simulink model "controller"  (Simulink 8.7)
settings: Solver=FixedStepAuto  StartTime=0.0  StopTime=10.0  FixedStep=0.01  RelTol=1e-3
settings Model: Creator=eispin  LastModifiedBy=max
settings DataIOCC: LimitDataPoints=off  SaveFormat=Dataset
settings DebuggingCC: UnderspecifiedInitializationDetection=Simplified  MergeDetectMultiDrivingBlocksExec=error
settings HardwareCC: ProdBitPerPointer=64  ProdLargestAtomicFloat=Float  ProdIntDivRoundTo=Zero  ProdEndianess=LittleEndian  ProdWordSize=64  ProdHWDeviceType=Intel->x86-64 (Windows64)
settings ModelReferenceCC: PropagateSignalLabelsOutOfModel=on
settings ConfigComp: CovModelRefEnable=off

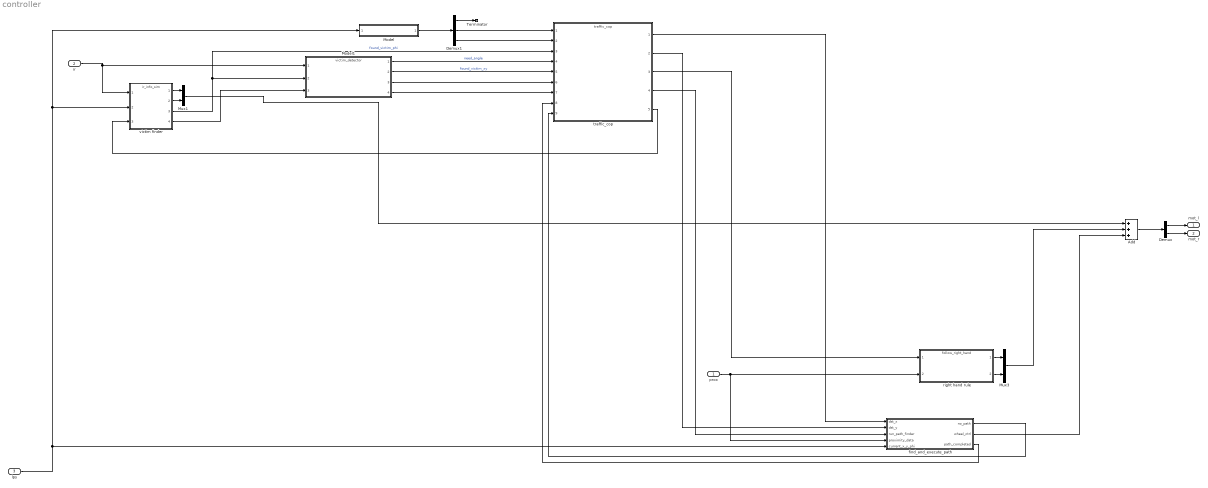
== system controller ==
  prox : Inport
  ir : Inport  Port=2
  lps : Inport  Port=3
  Add : Sum  Inputs=+++
  Demux : Demux  Outputs=2
  Demux1 : Demux  Outputs=3
  Model : ModelReference  ModelNameDialog=hold_initial  SimulationMode=Normal  ModelReferenceVersion=1.1
  Model1 : ModelReference  ModelNameDialog=victim_detector  SimulationMode=Normal  ModelReferenceVersion=1.2
  Mux1 : Mux  Inputs=2
  Mux3 : Mux  Inputs=2
  Terminator : Terminator
  find_and_execute_path : Subsystem
  right hand rule : ModelReference  ModelNameDialog=follow_right_hand.mdl  SimulationMode=Normal  ModelReferenceVersion=1.25
  traffic_cop : ModelReference  ModelNameDialog=traffic_cop  SimulationMode=Normal  ModelReferenceVersion=1.55
  victim finder : ModelReference  ModelNameDialog=ir_info_sim.slx  SimulationMode=Normal  ModelReferenceVersion=1.27
  mot_l : Outport
  mot_r : Outport  Port=2
  wires:
  lps/1 -> Model/1, victim finder/2, find_and_execute_path/5(current_x_y_phi)
  prox/1 -> find_and_execute_path/4(proximity_data), right hand rule/2
  ir/1 -> victim finder/1, Model1/1
  victim finder/3 -> traffic_cop/3, Model1/2  "found_victim_phi"
  victim finder/4 -> Model1/3
  Mux1/1 -> Add/1
  victim finder/2 -> Mux1/2
  victim finder/1 -> Mux1/1
  Mux3/1 -> Add/2
  right hand rule/2 -> Mux3/2
  right hand rule/1 -> Mux3/1
  Model/1 -> Demux1/1
  Model1/1 -> traffic_cop/4  "need_angle"
  Model1/2 -> traffic_cop/5  "found_victim_xy"
  traffic_cop/5 -> victim finder/3
  Model1/4 -> traffic_cop/7
  Demux1/3 -> traffic_cop/2
  Demux1/2 -> traffic_cop/1
  traffic_cop/3 -> right hand rule/1
  Model1/3 -> traffic_cop/6
  Demux1/1 -> Terminator/1
  Add/1 -> Demux/1
  Demux/1 -> mot_l/1
  Demux/2 -> mot_r/1
  traffic_cop/1 -> find_and_execute_path/1(dst_x)
  traffic_cop/2 -> find_and_execute_path/2(dst_y)
  traffic_cop/4 -> find_and_execute_path/3(run_path_finder)
  find_and_execute_path/1(no_path) -> traffic_cop/9
  find_and_execute_path/2(wheel_ctrl) -> Add/3
  find_and_execute_path/3(path_completed) -> traffic_cop/8

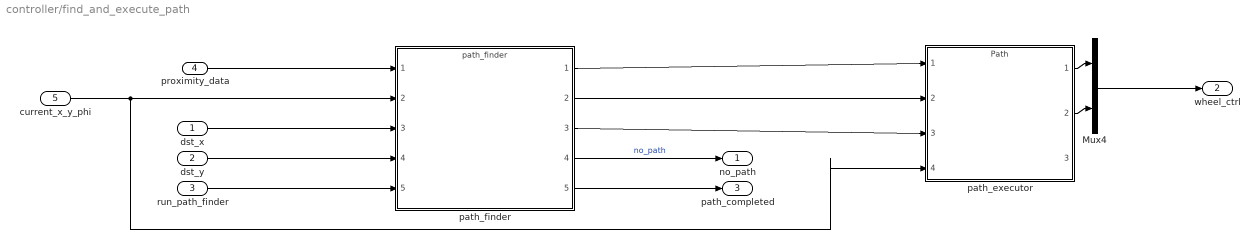
== system controller/find_and_execute_path ==
  dst_x : Inport
  dst_y : Inport  Port=2
  run_path_finder : Inport  Port=3
  proximity_data : Inport  Port=4
  current_x_y_phi : Inport  Port=5
  Mux4 : Mux  Inputs=2
  path_executor : ModelReference  ModelNameDialog=Path.slx  SimulationMode=Normal  ModelReferenceVersion=1.24
  path_finder : ModelReference  ModelNameDialog=path_finder  SimulationMode=Normal  ModelReferenceVersion=1.74
  no_path : Outport
  wheel_ctrl : Outport  Port=2
  path_completed : Outport  Port=3
  wires:
  proximity_data/1 -> path_finder/1
  current_x_y_phi/1 -> path_finder/2, path_executor/4
  path_finder/3 -> path_executor/3
  Mux4/1 -> wheel_ctrl/1
  dst_y/1 -> path_finder/4
  path_finder/4 -> no_path/1  "no_path"
  path_finder/2 -> path_executor/2
  path_finder/1 -> path_executor/1
  run_path_finder/1 -> path_finder/5
  path_executor/2 -> Mux4/2
  dst_x/1 -> path_finder/3
  path_executor/1 -> Mux4/1
  path_finder/5 -> path_completed/1
